simulink subsystem "Calculate_Prescribed_UFR"  (R2023a)
settings: Solver=VariableStepAuto  StartTime=0.0  StopTime=10.0  RelTol=1e-3
model mask{predw=73.2, postdw=70.6, dtime=4}
  mask prompts: predw "Pre-Dialysis Weight (kg)"; postdw "Post-Dialysis Weight (kg)"; dtime "Dialysis Treatment Time (hr)"
settings Model: Creator=ppatel  LastModifiedBy=ppatel

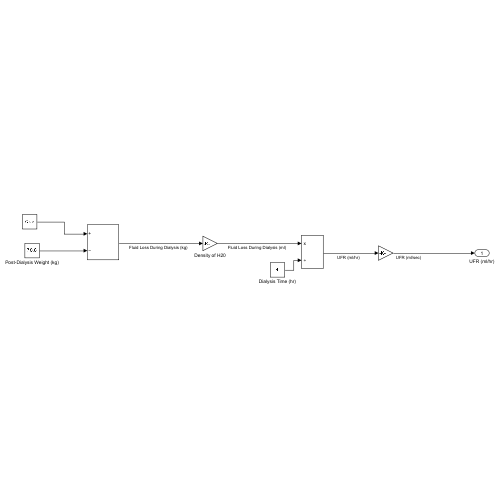
[thumbnail: Simulink's stored preview of the top-level diagram]
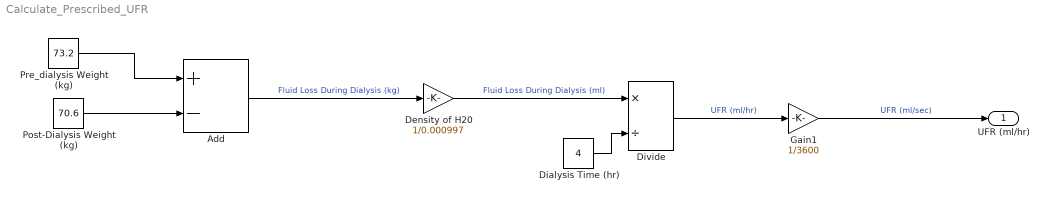
== system Calculate_Prescribed_UFR ==
  Add : Sum  Inputs=+-
  Density of H20 : Gain  Gain=1/0.000997
  Dialysis Time (hr) : Constant  Value=4
  Divide : Product  Inputs=*/
  Gain1 : Gain  Gain=1/3600
  Post-Dialysis Weight (kg) : Constant  Value=70.6
  Pre_dialysis Weight (kg) : Constant  Value=73.2
  UFR (ml/hr) : Outport
  wires:
  Add/1 -> Density of H20/1  "Fluid Loss During Dialysis (kg)"
  Divide/1 -> Gain1/1  "UFR (ml/hr)"
  Pre_dialysis Weight (kg)/1 -> Add/1
  Density of H20/1 -> Divide/1  "Fluid Loss During Dialysis (ml)"
  Post-Dialysis Weight (kg)/1 -> Add/2
  Dialysis Time (hr)/1 -> Divide/2
  Gain1/1 -> UFR (ml/hr)/1  "UFR (ml/sec)"
